simulink model "my_lqr"  (R2015a)
settings: Solver=ode4  StartTime=0.0  StopTime=1  FixedStep=0.01  RelTol=1e-3
values from neighbouring files (symbols this model uses):
  A_D = [1, 3; -0.5, 1]    [main.m]
  B_D = [0, 1]'    [main.m]
  x00 = [0.6, -0.7]'    [main.m]
undefined symbols (not defined in the file or in its folder): K
settings Model: Creator=andreas  LastModifiedBy=andreas

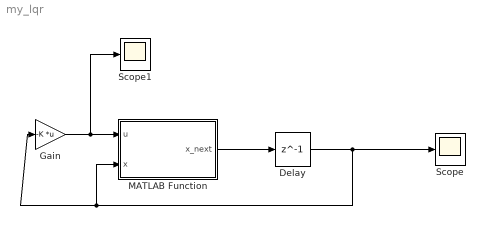
== system my_lqr ==
  Delay : Delay  DelayLength=1  InitialCondition=x00  SampleTime=0.01
  Gain : Gain  Gain=-K  Multiplication=Matrix(K*u)
  MATLAB Function : MATLAB Function  TreatAsAtomicUnit=on
  Scope : Scope
  Scope1 : Scope
  wires:
  MATLAB Function/1(x_next) -> Delay/1
  Gain/1 -> Scope1/1, MATLAB Function/1(u)
  Delay/1 -> MATLAB Function/2(x), Gain/1, Scope/1

== matlab function my_lqr/MATLAB Function ==
  data: u input; x input; x_next output; A_D parameter; B_D parameter
function x_next = fcn(u, x, A_D, B_D)
%#codegen
x_next = A_D*x + B_D*u;
